simulink model "Bldc_torque_control (1)"  (R2023a)
settings: Solver=FixedStepAuto  StartTime=0.0  StopTime=2  FixedStep=5e-7  RelTol=1e-3
undefined symbols (not defined in the file): sigbuilder_block
libraries: cstblocks x14, spsIGBTDiodeLib x12, spsCurrentMeasurementLib x8, spsSeriesRLCBranchLib x6, spsVoltageMeasurementLib x6, spsabctoAlphaBetaZeroLib x6, spsDCVoltageSourceLib x2, simulink x2, spsPermanentMagnetSynchronousMachineLib x2, spsTriangleGeneratorLib x2, spspowerguiLib x2
settings Model: Creator=kiran  LastModifiedBy=ANKIT

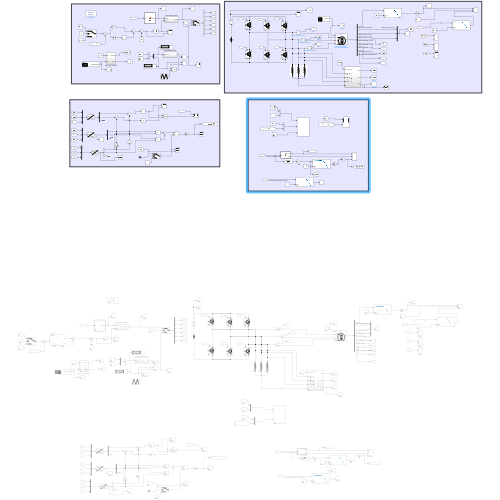
[thumbnail: Simulink's stored preview of the top-level diagram]
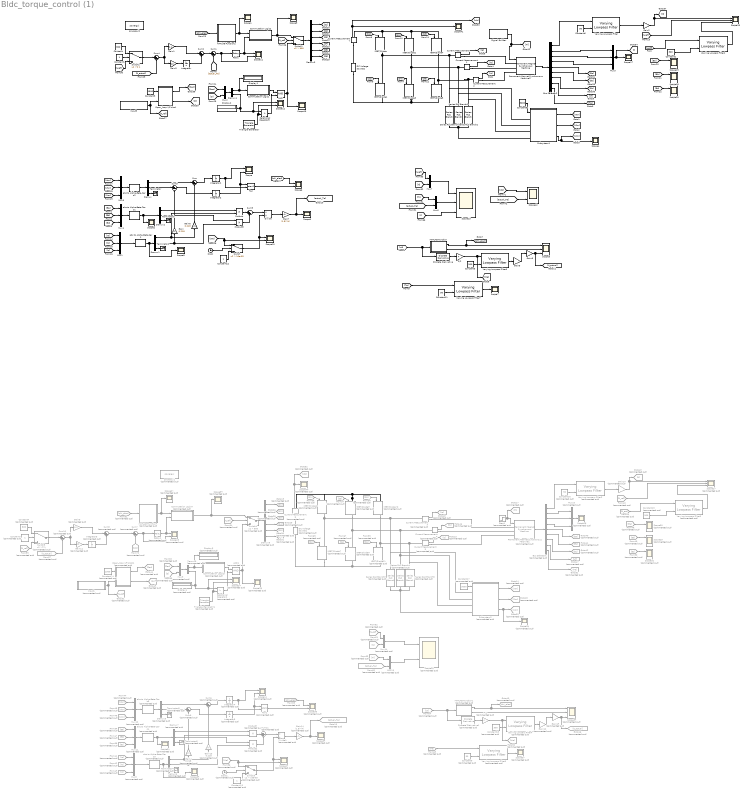
== system Bldc_torque_control (1) ==
  AND : Logic  IconShape=distinctive  AllPortsSameDT=off  OutDataTypeStr=boolean
  AND1 : Logic  Commented=on  IconShape=distinctive  AllPortsSameDT=off  OutDataTypeStr=boolean
  Bus Selector1 : BusSelector  Commented=on  OutputSignals=Rotor speed wm (rad/s),Stator current is_a (A),Stator current is_b (A),Stator current is_c (A),Stator back EMF e_a (V),Stator back EMF e_b (V),Stator back EMF e_cV),Rotor angle thetam (rad),Electromagnetic torque Te (N*m)
  Bus Selector2 : BusSelector  OutputSignals=Rotor speed wm (rad/s),Stator current is_a (A),Stator current is_b (A),Stator current is_c (A),Stator back EMF e_a (V),Stator back EMF e_b (V),Stator back EMF e_cV),Rotor angle thetam (rad),Electromagnetic torque Te (N*m)
  Clock : Clock
  Clock1 : Clock  Commented=on
  Commutation Logic1 : Subsystem
  Commutation Logic2 : Subsystem
  Commutation Logic3 : Subsystem  Commented=on
  Commutation Logic4 : Subsystem  Commented=on
  Constant : Constant  Value=800
  Constant1 : Constant
  Constant10 : Constant  Commented=on
  Constant11 : Constant  Value=50
  Constant12 : Constant
  Constant13 : Constant  Commented=on  Value=300
  Constant14 : Constant  Commented=on  Value=1500
  Constant15 : Constant  Commented=on  Value=300
  Constant16 : Constant  Commented=on  Value=50
  Constant17 : Constant  Commented=on  Value=3000
  Constant2 : Constant  Value=300
  Constant3 : Constant  Value=1500
  Constant4 : Constant  Commented=on  Value=800
  Constant5 : Constant  Value=300
  Constant6 : Constant  Value=50
  Constant7 : Constant  Commented=on
  Constant8 : Constant  Value=3000
  Constant9 : Constant  Commented=on  Value=50
  Current Measurement{,1..2,7} (4 alike) : spsCurrentMeasurementLib/Current Measurement  PhasorSimulation=off  OutputType=Complex  PSBequivalent=0
  Current Measurement{3..6} (4 alike) : spsCurrentMeasurementLib/Current Measurement  Commented=on  PhasorSimulation=off  OutputType=Complex  PSBequivalent=0
  DC Voltage Source1 : spsDCVoltageSourceLib/DC Voltage Source  Commented=on  Amplitude=33  Measurements=None
  DC Voltage Source2 : spsDCVoltageSourceLib/DC Voltage Source  Amplitude=33  Measurements=None
  Demux : Demux  Outputs=3
  Demux1 : Demux  Outputs=3
  Demux2 : Demux  Outputs=3
  Demux3 : Demux  Outputs=6
  Demux4 : Demux  Outputs=2
  Demux5 : Demux  Commented=on  Outputs=3
  Demux6 : Demux  Commented=on  Outputs=3
  Demux7 : Demux  Commented=on  Outputs=3
  Demux8 : Demux  Commented=on  Outputs=6
  Demux9 : Demux  Commented=on  Outputs=2
  Discrete Derivative : simulink/Discrete/Discrete Derivative  gainval=1.0  ICPrevScaledInput=0.0  OutMin=[]  OutMax=[]  OutDataType=fixdt(1, 16)  OutScaling=2^-10  DoSatur=off
  Discrete Derivative1 : simulink/Discrete/Discrete Derivative  Commented=on  gainval=1.0  ICPrevScaledInput=0.0  OutMin=[]  OutMax=[]  OutDataType=fixdt(1, 16)  OutScaling=2^-10  DoSatur=off
  Display1 : Display
  Display2 : Display
  Display3 : Display  Commented=on
  Display4 : Display  Commented=on
  Divide : Product  Inputs=*/
  Divide1 : Product  Commented=on  Inputs=*/
  From35 : From  Commented=on  GotoTag=N_est
  From36 : From  Commented=on  GotoTag=Ea
  From37 : From  Commented=on  GotoTag=S3
  From38 : From  Commented=on  GotoTag=S5
  From39 : From  Commented=on  GotoTag=S6
  From{40,54,59,62} (4 alike) : From  Commented=on  GotoTag=N_ref
  From41 : From  Commented=on  GotoTag=Ia
  From42 : From  Commented=on  GotoTag=Ib
  From43 : From  Commented=on  GotoTag=Ic
  From44 : From  Commented=on  GotoTag=Van
  From45 : From  Commented=on  GotoTag=Vbn
  From46 : From  Commented=on  GotoTag=Vcn
  From47 : From  Commented=on  GotoTag=Eb
  From48 : From  Commented=on  GotoTag=Ea
  From49 : From  Commented=on  GotoTag=Eb
  From50 : From  Commented=on  GotoTag=Ec
  From51 : From  Commented=on  GotoTag=phi_elec
  From52 : From  Commented=on  GotoTag=Sec
  From53 : From  Commented=on  GotoTag=D
  From55 : From  Commented=on  GotoTag=phi_elec
  From56 : From  Commented=on  GotoTag=We
  From57 : From  Commented=on  GotoTag=N_actual
  From58 : From  Commented=on  GotoTag=Ec
  From60 : From  Commented=on  GotoTag=actual_Te
  From61 : From  Commented=on  GotoTag=N
  From63 : From  Commented=on  GotoTag=Tl
  From64 : From  Commented=on  GotoTag=wt
  From65 : From  Commented=on  GotoTag=Te
  From67 : From  Commented=on  GotoTag=S4
  From68 : From  Commented=on  GotoTag=S1
  From69 : From  Commented=on  GotoTag=S2
  From70 : From  Commented=on  GotoTag=Idc
  Gain : Gain  Gain=0.218
  Gain1 : Gain  Gain=0.1
  Gain10 : Gain  Commented=on  Gain=30/pi
  Gain11 : Gain  Commented=on  Gain=10
  Gain12 : Gain  Commented=on  Gain=30/pi
  Gain13 : Gain  Commented=on  Gain=0.218
  Gain14 : Gain  Commented=on  Gain=(1.5)*(4)
  Gain15 : Gain  Commented=on  Gain=0.25
  Gain2 : Gain  Gain=30/pi
  Gain3 : Gain  Gain=10
  Gain4 : Gain  Commented=on  Gain=0.218
  Gain5 : Gain  Gain=30/pi
  Gain6 : Gain  Gain=0.218
  Gain7 : Gain  Gain=(1.5)*(4)
  Gain8 : Gain  Gain=0.25
  Gain9 : Gain  Commented=on  Gain=0.1
  Goto13 : Goto  Commented=on  GotoTag=Ic
  Goto14 : Goto  Commented=on  GotoTag=Van
  Goto15 : Goto  Commented=on  GotoTag=actual_Te
  Goto16 : Goto  Commented=on  GotoTag=N_actual
  Goto17 : Goto  Commented=on  GotoTag=Tl
  Goto18 : Goto  Commented=on  GotoTag=Vbn
  Goto19 : Goto  Commented=on  GotoTag=S1
  Goto26 : Goto  Commented=on  GotoTag=S2
  Goto28 : Goto  Commented=on  GotoTag=S3
  Goto29 : Goto  Commented=on  GotoTag=S4
  Goto30 : Goto  Commented=on  GotoTag=S5
  Goto31 : Goto  Commented=on  GotoTag=S6
  Goto32 : Goto  Commented=on  GotoTag=N_ref
  Goto33 : Goto  Commented=on  GotoTag=Vcn
  Goto40 : Goto  Commented=on  GotoTag=Ea
  Goto41 : Goto  Commented=on  GotoTag=Eb
  Goto42 : Goto  Commented=on  GotoTag=Ec
  Goto43 : Goto  Commented=on  GotoTag=N
  Goto44 : Goto  Commented=on  GotoTag=Sec
  Goto45 : Goto  Commented=on  GotoTag=D
  Goto46 : Goto  Commented=on  GotoTag=Ib
  Goto47 : Goto  Commented=on  GotoTag=wt
  Goto48 : Goto  Commented=on  GotoTag=Ia
  Goto49 : Goto  Commented=on  GotoTag=phi_elec
  Goto50 : Goto  Commented=on  GotoTag=We
  Goto51 : Goto  Commented=on  GotoTag=Te
  Goto52 : Goto  Commented=on  GotoTag=Idc
  IGBT/Diode{,1..5} (6 alike) : spsIGBTDiodeLib/IGBT//Diode  Ron=1e-3  Rs=1e5  Cs=inf  Measurements=on
  IGBT/Diode{6..11} (6 alike) : spsIGBTDiodeLib/IGBT//Diode  Commented=on  Ron=1e-3  Rs=1e5  Cs=inf  Measurements=on
  Input1 : Subsystem  Tag=STV Subsys  Commented=on  LoadFcn=sigbuilder_block('load');  StartFcn=sigbuilder_block('start');  StopFcn=sigbuilder_block('stop');  ClipboardFcn=sigbuilder_block('clipboard');  mask(Sigbuilder block){tuvar=[0:10]}
      mask help: Simulink:masks:SigbuilderBlock_MD
      mask init:
      | if ~strcmp(get_param(bdroot(gcbh),'SimulationStatus'),'stopped') tuvar = sigbuilder_block('maskInit'); end
      settings: CopyFcn=sigbuilder_block('copy');  DeleteFcn=sigbuilder_block('delete');  ModelCloseFcn=sigbuilder_block('modelClose');  PreSaveFcn=sigbuilder_block('preSave');  PauseFcn=sigbuilder_block('pause');  ContinueFcn=sigbuilder_block('continue');  NameChangeFcn=sigbuilder_block('namechange');  OpenFcn=sigbuilder_block('open',[6 36 1524 722.25 ]);  CloseFcn=sigbuilder_block('close');
      mask Display: plot(0, 0, 100, 100,[2, 2, 32, 32, 2], [68, 8, 8, 68, 68],[32, 2], [38, 38], [32, 19, 2],[53, 60, 44], [32, 17, 17, 2],[16, 16, 31, 31]);txt = getActiveGroup(gcbh);text(2, 100, txt,'verticalAlignment', 'top');
  Input3 : Subsystem  Tag=STV Subsys  LoadFcn=sigbuilder_block('load');  StartFcn=sigbuilder_block('start');  StopFcn=sigbuilder_block('stop');  ClipboardFcn=sigbuilder_block('clipboard');  mask(Sigbuilder block){tuvar=[0:10]}
      mask help: Simulink:masks:SigbuilderBlock_MD
      mask init:
      | if ~strcmp(get_param(bdroot(gcbh),'SimulationStatus'),'stopped') tuvar = sigbuilder_block('maskInit'); end
      settings: CopyFcn=sigbuilder_block('copy');  DeleteFcn=sigbuilder_block('delete');  ModelCloseFcn=sigbuilder_block('modelClose');  PreSaveFcn=sigbuilder_block('preSave');  PauseFcn=sigbuilder_block('pause');  ContinueFcn=sigbuilder_block('continue');  NameChangeFcn=sigbuilder_block('namechange');  OpenFcn=sigbuilder_block('open',[6 36 1524 722.25 ]);  CloseFcn=sigbuilder_block('close');
      mask Display: plot(0, 0, 100, 100,[2, 2, 32, 32, 2], [68, 8, 8, 68, 68],[32, 2], [38, 38], [32, 19, 2],[53, 60, 44], [32, 17, 17, 2],[16, 16, 31, 31]);txt = getActiveGroup(gcbh);text(2, 100, txt,'verticalAlignment', 'top');
  Integrator : Integrator
  Integrator1 : Integrator
  Integrator2 : Integrator
  Integrator3 : Integrator  Commented=on
  Integrator4 : Integrator  Commented=on
  Integrator5 : Integrator  Commented=on
  MATLAB Function : MATLAB Function  TreatAsAtomicUnit=on
  MATLAB Function1 : MATLAB Function  Commented=on  TreatAsAtomicUnit=on
  MATLAB Function2 : MATLAB Function  TreatAsAtomicUnit=on
  MATLAB Function3 : MATLAB Function  Commented=on  TreatAsAtomicUnit=on
  Mux{1,3..5} (4 alike) : Mux  Inputs=3
  Mux{8,10..12} (4 alike) : Mux  Commented=on  Inputs=3
  Mux13 : Mux  Commented=on  Inputs=2
  Mux14 : Mux  Commented=on  Inputs=2
  Mux2 : Mux  Inputs=2
  Mux6 : Mux  Inputs=2
  Mux7 : Mux  Inputs=2
  Mux9 : Mux  Commented=on  Inputs=2
  Open_loop V/f block : Subsystem
  Open_loop V/f block1 : Subsystem  Commented=on
  P/1 : Gain  Commented=on  Gain=4
  P/2 : Gain  Gain=4
  Permanent Magnet Synchronous Machine1 : spsPermanentMagnetSynchronousMachineLib/Permanent Magnet Synchronous Machine  Commented=on  NbPhases=3  FluxDistribution=Trapezoidal  RotorType=Round  MechanicalLoad=Torque Tm  PresetModel="05:  8 Nm 300 Vdc 2000 RPM - 10 Nm"  ShowDetailedParameters=on  MeasurementBus=off  Resistance=0.218  Inductance=0.264e-3  dqInductances=[0.0133 0.0147]  La=0.00525  MachineConstant=Voltage Constant (V_peak L-L / krpm)  Flux=0.0188  VoltageCst=15.7499  TorqueCst=0.1504  Flat=120  Mechanical=[0.00028 0.0003035 4 0]  PolePairs=4  InitialConditions=[0,0, 0,0]  InitialConditions5ph=[0 0 0 0 0 0]  RefAngle=Aligned with phase A axis (original Park)  IterativeDiscreteModel=Trapezoidal non iterative  TsBlock=-1  TsPowergui=0
  Permanent Magnet Synchronous Machine2 : spsPermanentMagnetSynchronousMachineLib/Permanent Magnet Synchronous Machine  NbPhases=3  FluxDistribution=Trapezoidal  RotorType=Round  MechanicalLoad=Torque Tm  PresetModel="05:  8 Nm 300 Vdc 2000 RPM - 10 Nm"  ShowDetailedParameters=on  MeasurementBus=off  Resistance=0.218  Inductance=0.264e-3  dqInductances=[0.0133 0.0147]  La=0.00525  MachineConstant=Voltage Constant (V_peak L-L / krpm)  Flux=0.0188  VoltageCst=15.7499  TorqueCst=0.1504  Flat=120  Mechanical=[0.00028 0.0003035 4 0]  PolePairs=4  InitialConditions=[0,0, 0,0]  InitialConditions5ph=[0 0 0 0 0 0]  RefAngle=Aligned with phase A axis (original Park)  IterativeDiscreteModel=Trapezoidal non iterative  TsBlock=-1  TsPowergui=0
  Product : Product
  Product1 : Product  Commented=on
  Product2 : Product  Commented=on
  Product3 : Product
  Relational Operator1 : RelationalOperator  Commented=on  Operator=>  OutDataTypeStr=boolean  RndMeth=Simplest  InputSameDT=off
  Relational Operator3 : RelationalOperator  Operator=>  OutDataTypeStr=boolean  RndMeth=Simplest  InputSameDT=off
  Relay : Relay  OnSwitchValue=0.05  OffSwitchValue=-0.05  OffOutputValue=-1
  Relay1 : Relay  Commented=on  OnSwitchValue=0.1  OffSwitchValue=-0.1  OffOutputValue=-1
  Scope{,6,10..12,19..20,42} (8 alike) : Scope  NumInputPorts=2
  Scope{1..2,4..5,7..9,15,17,41} (10 alike) : Scope
  Scope{3,13,16,18} (4 alike) : Scope  NumInputPorts=3
  Scope{14,22..25,30,32,36} (8 alike) : Scope  Commented=on  NumInputPorts=2
  Scope{21,26,28,31,34..35,37..40} (10 alike) : Scope  Commented=on
  Scope27 : Scope  Commented=on  NumInputPorts=3
  Scope29 : Scope  Commented=on  NumInputPorts=3
  Scope33 : Scope  Commented=on  NumInputPorts=3
  Series RLC Branch : spsSeriesRLCBranchLib/Series RLC Branch  LConnTagsString=__new0  RConnTagsString=__new0  BranchType=R  Resistance=1e06  Inductance=1e-3  SetiL0=off  InitialCurrent=0  Capacitance=1e-6  Setx0=off  InitialVoltage=0  Measurements=None
  Series RLC Branch1 : spsSeriesRLCBranchLib/Series RLC Branch  LConnTagsString=__new0  RConnTagsString=__new0  BranchType=R  Resistance=1e06  Inductance=1e-3  SetiL0=off  InitialCurrent=0  Capacitance=1e-6  Setx0=off  InitialVoltage=0  Measurements=None
  Series RLC Branch2 : spsSeriesRLCBranchLib/Series RLC Branch  LConnTagsString=__new0  RConnTagsString=__new0  BranchType=R  Resistance=1e06  Inductance=1e-3  SetiL0=off  InitialCurrent=0  Capacitance=1e-6  Setx0=off  InitialVoltage=0  Measurements=None
  Series RLC Branch3 : spsSeriesRLCBranchLib/Series RLC Branch  Commented=on  LConnTagsString=__new0  RConnTagsString=__new0  BranchType=R  Resistance=1e06  Inductance=1e-3  SetiL0=off  InitialCurrent=0  Capacitance=1e-6  Setx0=off  InitialVoltage=0  Measurements=None
  Series RLC Branch4 : spsSeriesRLCBranchLib/Series RLC Branch  Commented=on  LConnTagsString=__new0  RConnTagsString=__new0  BranchType=R  Resistance=1e06  Inductance=1e-3  SetiL0=off  InitialCurrent=0  Capacitance=1e-6  Setx0=off  InitialVoltage=0  Measurements=None
  Series RLC Branch5 : spsSeriesRLCBranchLib/Series RLC Branch  Commented=on  LConnTagsString=__new0  RConnTagsString=__new0  BranchType=R  Resistance=1e06  Inductance=1e-3  SetiL0=off  InitialCurrent=0  Capacitance=1e-6  Setx0=off  InitialVoltage=0  Measurements=None
  Signal Builder : Subsystem  Tag=STV Subsys  LoadFcn=sigbuilder_block('load');  StartFcn=sigbuilder_block('start');  StopFcn=sigbuilder_block('stop');  ClipboardFcn=sigbuilder_block('clipboard');  mask(Sigbuilder block){tuvar=[0:10]}
      mask help: Simulink:masks:SigbuilderBlock_MD
      mask init:
      | if ~strcmp(get_param(bdroot(gcbh),'SimulationStatus'),'stopped') tuvar = sigbuilder_block('maskInit'); end
      settings: CopyFcn=sigbuilder_block('copy');  DeleteFcn=sigbuilder_block('delete');  ModelCloseFcn=sigbuilder_block('modelClose');  PreSaveFcn=sigbuilder_block('preSave');  PauseFcn=sigbuilder_block('pause');  ContinueFcn=sigbuilder_block('continue');  NameChangeFcn=sigbuilder_block('namechange');  OpenFcn=sigbuilder_block('open',[0 36 1536 766.5 ]);  CloseFcn=sigbuilder_block('close');
      mask Display: plot(0, 0, 100, 100,[2, 2, 32, 32, 2], [68, 8, 8, 68, 68],[32, 2], [38, 38], [32, 19, 2],[53, 60, 44], [32, 17, 17, 2],[16, 16, 31, 31]);txt = getActiveGroup(gcbh);text(2, 100, txt,'verticalAlignment', 'top');
  Step1 : Step  Commented=on  After=0.8  SampleTime=0
  Subsystem1 : Subsystem
  Subsystem2 : Subsystem  Commented=on
  Sum{,1,3..4} (4 alike) : Sum  Inputs=|+-
  Sum{6..7,9..10} (4 alike) : Sum  Commented=on  Inputs=|+-
  Sum11 : Sum  Commented=on  Inputs=|++
  Sum2 : Sum  Inputs=|++
  Sum5 : Sum  Inputs=|++
  Sum8 : Sum  Commented=on  Inputs=|++
  Switch : Switch  Criteria=u2 > Threshold  Threshold=10e-03  SaturateOnIntegerOverflow=off  InputSameDT=off
  Switch1 : Switch  Criteria=u2 > Threshold  Threshold=900  SaturateOnIntegerOverflow=off  InputSameDT=off
  Switch2 : Switch  Threshold=1  SaturateOnIntegerOverflow=off  InputSameDT=off
  Switch3 : Switch  Commented=on  Criteria=u2 > Threshold  Threshold=10e-03  SaturateOnIntegerOverflow=off  InputSameDT=off
  Switch4 : Switch  Commented=on  Criteria=u2 > Threshold  Threshold=900  SaturateOnIntegerOverflow=off  InputSameDT=off
  Switch5 : Switch  Commented=on  Threshold=1  SaturateOnIntegerOverflow=off  InputSameDT=off
  Tan : Trigonometry  Operator=atan2
  Tan1 : Trigonometry  Commented=on  Operator=atan2
  Terminator : Terminator
  Terminator1 : Terminator
  Terminator2 : Terminator
  Terminator3 : Terminator  Commented=on
  Terminator4 : Terminator  Commented=on
  Terminator5 : Terminator  Commented=on
  Triangle Generator : spsTriangleGeneratorLib/Triangle Generator  Freq=10e3  Phase=0  Ts=0
  Triangle Generator1 : spsTriangleGeneratorLib/Triangle Generator  Commented=on  Freq=10e3  Phase=0  Ts=0
  Varying Lowpass Filter{,1,6..7} (4 alike) : cstblocks/Linear Parameter Varying/Varying Lowpass Filter  N=1
  Varying Lowpass Filter{2..5} (4 alike) : cstblocks/Linear Parameter Varying/Varying Lowpass Filter  Commented=on  N=1
  abc to Alpha-Beta-Zero : spsabctoAlphaBetaZeroLib/abc to Alpha-Beta-Zero
  abc to Alpha-Beta-Zero1 : spsabctoAlphaBetaZeroLib/abc to Alpha-Beta-Zero
  abc to Alpha-Beta-Zero2 : spsabctoAlphaBetaZeroLib/abc to Alpha-Beta-Zero
  abc to Alpha-Beta-Zero3 : spsabctoAlphaBetaZeroLib/abc to Alpha-Beta-Zero  Commented=on
  abc to Alpha-Beta-Zero4 : spsabctoAlphaBetaZeroLib/abc to Alpha-Beta-Zero  Commented=on
  abc to Alpha-Beta-Zero5 : spsabctoAlphaBetaZeroLib/abc to Alpha-Beta-Zero  Commented=on
  powergui1 : spspowerguiLib/powergui  Priority=1  Commented=on  SimulationMode=Discrete  SampleTime=1e-6  frequency=60  Iterations=50  frequencyindice=0  Pbase=100e6  ErrMax=1e-4  UnitsV=kV  UnitsW=MW  buscounter=0  FunctionMessages=off  echomessages=off  EnableUseOfTLC=off  CurrentSourceSwitches=off  DisableSnubberDevices=off  DisableRonSwitches=off  DisableVfSwitches=off  DisplayEquations=off  AutomaticDiscreteSolvers=off  SolverType=Tustin/Backward Euler (TBE)  Interpol=off  ExternalGateDelay=off  methode=off  Ts=100  x0status=blocks  SPID=on  SwTol=0  HookPort=off  NonlinearTolerance=1e-4  nMaxIteration=100  ContinueOnMaxIteration=off  RestoreLinks=warning  ResistiveCurrentMeasurement=off  Frange=[0:2:500]  Ylog=off  Xlog=on  ShowGrid=off  save=off  variable=ZData  structure=0  ZoomFFT=off  StartTime=0.0  cycles=1  DisplayStyle=1  fundamental=60  FreqAxis=off  MaxFrequency=1000  frequencyindicesteady=1  RmsSteady=1  display=off
  powergui2 : spspowerguiLib/powergui  Priority=1  SimulationMode=Discrete  SampleTime=1e-6  frequency=60  Iterations=50  frequencyindice=0  Pbase=100e6  ErrMax=1e-4  UnitsV=kV  UnitsW=MW  buscounter=0  FunctionMessages=off  echomessages=off  EnableUseOfTLC=off  CurrentSourceSwitches=off  DisableSnubberDevices=off  DisableRonSwitches=off  DisableVfSwitches=off  DisplayEquations=off  AutomaticDiscreteSolvers=off  SolverType=Tustin/Backward Euler (TBE)  Interpol=off  ExternalGateDelay=off  methode=off  Ts=100  x0status=blocks  SPID=on  SwTol=0  HookPort=off  NonlinearTolerance=1e-4  nMaxIteration=100  ContinueOnMaxIteration=off  RestoreLinks=warning  ResistiveCurrentMeasurement=off  Frange=[0:2:500]  Ylog=off  Xlog=on  ShowGrid=off  save=off  variable=ZData  structure=0  ZoomFFT=off  StartTime=0.0  cycles=1  DisplayStyle=1  fundamental=60  FreqAxis=off  MaxFrequency=1000  frequencyindicesteady=1  RmsSteady=1  display=off
  wires:
  [S1] -> IGBT/Diode/1
  Bus Selector2/3 -> Mux3/2  "<Stator current is_b (A)>"
  [Ec] -> Scope20/1
  [S5] -> IGBT/Diode4/1
  Permanent Magnet Synchronous Machine2/1 -> Bus Selector2/1
  [S2] -> IGBT/Diode1/1
  [S4] -> IGBT/Diode3/1
  Bus Selector2/2 -> Mux3/1  "<Stator current is_a (A)>"
  Constant6/1 -> Varying Lowpass Filter/2
  Bus Selector2/1 -> Varying Lowpass Filter/1  "<Rotor speed wm (rad/s)>"
  Mux3/1 -> [I], Scope17/1
  Bus Selector2/4 -> Mux3/3  "<Stator current is_c (A)>"
  Varying Lowpass Filter/1 -> Gain2/1
  Gain2/1 -> [N], Scope16/1
  [S6] -> IGBT/Diode5/1
  [Ea] -> Scope19/1
  [Eb] -> Scope18/1
  Bus Selector2/6 -> [Eb]  "<Stator back EMF e_b (V)>"
  [S3] -> IGBT/Diode2/1
  Bus Selector2/5 -> [Ea]  "<Stator back EMF e_a (V)>"
  Bus Selector2/7 -> [Ec]  "<Stator back EMF e_cV)>"
  [N_ref] -> Scope16/2
  Constant2/1 -> Varying Lowpass Filter1/2
  Varying Lowpass Filter1/1 -> Scope16/3
  [N_est] -> Varying Lowpass Filter1/1
  [Ea] -> Mux4/1
  [Eb] -> Mux4/2
  [Ec] -> Mux4/3
  Mux4/1 -> abc to Alpha-Beta-Zero1/1
  Bus Selector2/8 -> [wt]  "<Rotor angle thetam (rad)>"
  Subsystem1/2(Vbn) -> [Vbn]
  Constant8/1 -> Subsystem1/1(Cut_off_freq)
  Subsystem1/1(Van) -> [Van]
  Subsystem1/3(Vcn) -> Scope4/1, [Vcn]
  Current Measurement2/1 -> [Ic]
  Current Measurement1/1 -> [Ib]
  Current Measurement/1 -> [Ia]
  [Ia] -> Mux1/1
  Mux1/1 -> abc to Alpha-Beta-Zero/1
  [Ib] -> Mux1/2
  [Ic] -> Mux1/3
  [Vbn] -> Mux5/2
  Mux5/1 -> abc to Alpha-Beta-Zero2/1
  [Van] -> Mux5/1
  [Vcn] -> Mux5/3
  abc to Alpha-Beta-Zero2/1 -> Demux/1
  Demux/3 -> Terminator/1
  Demux/1 -> Sum/1
  Demux/2 -> Sum3/1
  Demux1/3 -> Terminator1/1
  Demux1/2 -> Product3/2, Gain/1
  Gain6/1 -> Sum/2
  Demux1/1 -> Product/2, Gain6/1
  Sum/1 -> Integrator1/1
  Sum3/1 -> Integrator2/1
  [phi_elec] -> Scope6/1
  Tan/1 -> Scope6/2
  Demux2/2 -> Product3/1
  abc to Alpha-Beta-Zero1/1 -> Demux2/1, Scope2/1
  Demux2/3 -> Terminator2/1
  Demux2/1 -> Product/1
  Product/1 -> Sum5/1
  Product3/1 -> Sum5/2
  Sum5/1 -> Divide/1
  Divide/1 -> Gain7/1
  Bus Selector2/9 -> [Te]  "<Electromagnetic torque Te (N*m)>"
  [We] -> Scope10/2, Switch/1
  Switch/1 -> Scope10/1, Divide/2
  Clock/1 -> Switch/2
  Constant12/1 -> Switch/3
  Gain7/1 -> Scope5/1, [actual_Te]
  abc to Alpha-Beta-Zero/1 -> Scope8/1, Demux1/1
  Sum2/1 -> Sum1/1
  [actual_Te] -> Sum1/2
  Sum1/1 -> Scope11/2, Relay/1
  Relay/1 -> Commutation Logic2/2(Tau), Scope11/1
  [phi_elec] -> MATLAB Function2/1(wt)
  MATLAB Function2/1(sector) -> Commutation Logic2/1(sector), Scope1/1
  Commutation Logic2/1(pulses) -> Scope9/1, Switch1/1
  Demux3/5 -> [S5]
  Demux3/2 -> [S2]
  Demux3/1 -> [S1]
  Demux3/3 -> [S3]
  Demux3/4 -> [S4]
  Switch1/1 -> Demux3/1
  Demux3/6 -> [S6]
  Demux4/1 -> Display1/1, Commutation Logic1/1(sector)
  Input3/1(RpmRequest) -> Open_loop V/f block/2(Wr), [N_ref]
  Commutation Logic1/1(Out1) -> AND/1
  [Sec] -> Mux2/1
  [D] -> Mux2/2
  Open_loop V/f block/2(Duty) -> [D]
  Open_loop V/f block/1(Sector) -> [Sec]
  Mux2/1 -> Demux4/1
  Constant3/1 -> Open_loop V/f block/1(Ws)
  Relational Operator3/1 -> AND/2
  AND/1 -> Scope15/1, Switch1/3
  Triangle Generator/1 -> Scope12/2, Relational Operator3/2
  Demux4/2 -> Display2/1, Scope12/1, Relational Operator3/1
  [N_ref] -> Switch1/2
  Integrator1/1 -> Tan/2, Scope/1
  Gain/1 -> Sum3/2
  Integrator2/1 -> Scope/2, Tan/1
  Varying Lowpass Filter7/1 -> Scope7/1
  [Te] -> Varying Lowpass Filter7/1
  Constant5/1 -> Varying Lowpass Filter6/2
  Gain8/1 -> [N_actual], Scope3/3
  MATLAB Function/2(phi) -> Scope3/2
  Discrete Derivative/1 -> P/2/1
  [wt] -> Discrete Derivative/1, MATLAB Function/1(wt)
  MATLAB Function/1(phi_elec) -> [phi_elec], Scope3/1
  Varying Lowpass Filter6/1 -> Gain5/1
  Constant11/1 -> Varying Lowpass Filter7/2
  P/2/1 -> [We], Varying Lowpass Filter6/1
  Gain5/1 -> Gain8/1
  Signal Builder/1(Signal 1) -> Permanent Magnet Synchronous Machine2/1, [Tl]
  Integrator/1 -> Sum2/2
  Gain1/1 -> Sum2/1
  [N_ref] -> Switch2/3
  Constant1/1 -> Switch2/2
  Constant/1 -> Switch2/1
  Gain3/1 -> Integrator/1
  Switch2/1 -> Sum4/1
  Sum4/1 -> Gain3/1, Gain1/1
  [N_actual] -> Sum4/2
  [actual_Te] -> Mux6/2
  [Tl] -> Mux6/1
  Mux7/1 -> Scope13/1
  Mux6/1 -> Scope13/2
  [N] -> Mux7/2
  [N_ref] -> Mux7/1
  From61/1 -> Mux14/2
  From63/1 -> Mux13/1
  Mux14/1 -> Scope25/1
  From57/1 -> Sum10/2
  Sum10/1 -> Gain11/1, Gain9/1
  Step1/1 -> Goto17/1, Permanent Magnet Synchronous Machine1/1
  Gain12/1 -> Gain15/1
  Constant7/1 -> Switch5/2
  Constant4/1 -> Switch5/1
  Demux6/3 -> Terminator4/1
  Gain11/1 -> Integrator3/1
  From55/1 -> Scope36/1
  Discrete Derivative1/1 -> P/1/1
  Mux11/1 -> abc to Alpha-Beta-Zero4/1
  MATLAB Function1/2(phi) -> Scope33/2
  Switch5/1 -> Sum10/1
  Divide1/1 -> Gain14/1
  From59/1 -> Switch5/3
  Gain9/1 -> Sum8/1
  Sum7/1 -> Scope23/2, Relay1/1
  abc to Alpha-Beta-Zero5/1 -> Demux5/1
  Demux8/6 -> Goto31/1
  AND1/1 -> Scope26/1, Switch4/3
  From51/1 -> MATLAB Function3/1(wt)
  Varying Lowpass Filter5/1 -> Scope37/1
  Demux9/2 -> Display4/1, Scope24/1, Relational Operator1/1
  P/1/1 -> Goto50/1, Varying Lowpass Filter4/1
  From64/1 -> Discrete Derivative1/1, MATLAB Function1/1(wt)
  Demux6/1 -> Product1/2, Gain13/1
  Integrator3/1 -> Sum8/2
  From60/1 -> Mux13/2
  Constant17/1 -> Subsystem2/1(Cut_off_freq)
  Bus Selector1/6 -> Goto41/1  "<Stator back EMF e_b (V)>"
  Relay1/1 -> Commutation Logic4/2(Tau), Scope23/1
  Integrator5/1 -> Scope14/2, Tan1/1
  From65/1 -> Varying Lowpass Filter5/1
  Open_loop V/f block1/2(Duty) -> Goto45/1
  From54/1 -> Switch4/2
  Gain13/1 -> Sum6/2
  Triangle Generator1/1 -> Scope24/2, Relational Operator1/2
  Varying Lowpass Filter4/1 -> Gain12/1
  Commutation Logic3/1(Out1) -> AND1/1
  Constant14/1 -> Open_loop V/f block1/1(Ws)
  Gain4/1 -> Sum9/2
  Product2/1 -> Sum11/2
  Demux8/1 -> Goto19/1
  Integrator4/1 -> Tan1/2, Scope14/1
  Varying Lowpass Filter2/1 -> Gain10/1
  From53/1 -> Mux9/2
  Input1/1(RpmRequest) -> Open_loop V/f block1/2(Wr), Goto32/1
  Commutation Logic4/1(pulses) -> Scope39/1, Switch4/1
  Bus Selector1/3 -> Mux10/2  "<Stator current is_b (A)>"
  Demux8/5 -> Goto30/1
  From69/1 -> IGBT/Diode7/1
  Switch4/1 -> Demux8/1
  From52/1 -> Mux9/1
  From35/1 -> Varying Lowpass Filter3/1
  From50/1 -> Scope32/1
  Demux9/1 -> Display3/1, Commutation Logic3/1(sector)
  From44/1 -> Mux12/1
  Open_loop V/f block1/1(Sector) -> Goto44/1
  Demux8/3 -> Goto28/1
  Sum11/1 -> Divide1/1
  Constant16/1 -> Varying Lowpass Filter2/2
  From36/1 -> Mux11/1
  From62/1 -> Mux14/1
  Gain14/1 -> Scope35/1, Goto15/1
  Bus Selector1/1 -> Varying Lowpass Filter2/1  "<Rotor speed wm (rad/s)>"
  Bus Selector1/4 -> Mux10/3  "<Stator current is_c (A)>"
  Varying Lowpass Filter3/1 -> Scope27/3
  From70/1 -> Sum7/2
  Sum8/1 -> Sum7/1
  Switch3/1 -> Scope22/1, Divide1/2
  Bus Selector1/9 -> Goto51/1  "<Electromagnetic torque Te (N*m)>"
  Demux7/1 -> Product1/1
  Constant13/1 -> Varying Lowpass Filter3/2
  abc to Alpha-Beta-Zero4/1 -> Demux7/1, Scope31/1
  From41/1 -> Mux8/1
  From42/1 -> Mux8/2
  Demux5/3 -> Terminator3/1
  Bus Selector1/5 -> Goto40/1  "<Stator back EMF e_a (V)>"
  Product1/1 -> Sum11/1
  Subsystem2/2(Vbn) -> Goto18/1
  From39/1 -> IGBT/Diode11/1
  From37/1 -> IGBT/Diode8/1
  Sum9/1 -> Integrator5/1
  Current Measurement3/1 -> Goto48/1
  From47/1 -> Mux11/2
  Sum6/1 -> Integrator4/1
  Demux6/2 -> Product2/2, Gain4/1
  Mux13/1 -> Scope25/2
  Demux7/2 -> Product2/1
  Mux12/1 -> abc to Alpha-Beta-Zero5/1
  From43/1 -> Mux8/3
  Tan1/1 -> Scope36/2
  MATLAB Function3/1(sector) -> Commutation Logic4/1(sector), Scope21/1
  Constant15/1 -> Varying Lowpass Filter4/2
  From45/1 -> Mux12/2
  Demux5/1 -> Sum6/1
  Current Measurement5/1 -> Goto13/1
  From49/1 -> Scope29/1
  Bus Selector1/7 -> Goto42/1  "<Stator back EMF e_cV)>"
  From58/1 -> Mux11/3
  From48/1 -> Scope30/1
  From40/1 -> Scope27/2
  Bus Selector1/8 -> Goto47/1  "<Rotor angle thetam (rad)>"
  Subsystem2/3(Vcn) -> Scope34/1, Goto33/1
  Demux5/2 -> Sum9/1
  Constant10/1 -> Switch3/3
  From68/1 -> IGBT/Diode6/1
  Demux7/3 -> Terminator5/1
  Mux8/1 -> abc to Alpha-Beta-Zero3/1
  Gain15/1 -> Goto16/1, Scope33/3
  Subsystem2/1(Van) -> Goto14/1
  Mux9/1 -> Demux9/1
  From56/1 -> Scope22/2, Switch3/1
  From38/1 -> IGBT/Diode10/1
  Mux10/1 -> Scope28/1
  Demux8/4 -> Goto29/1
  From67/1 -> IGBT/Diode9/1
  From46/1 -> Mux12/3
  Gain10/1 -> Goto43/1, Scope27/1
  abc to Alpha-Beta-Zero3/1 -> Scope38/1, Demux6/1
  Constant9/1 -> Varying Lowpass Filter5/2
  Clock1/1 -> Switch3/2
  Bus Selector1/2 -> Mux10/1  "<Stator current is_a (A)>"
  Relational Operator1/1 -> AND1/2
  Permanent Magnet Synchronous Machine1/1 -> Bus Selector1/1
  MATLAB Function1/1(phi_elec) -> Goto49/1, Scope33/1
  Current Measurement4/1 -> Goto46/1
  Demux8/2 -> Goto26/1
  Current Measurement6/1 -> Goto52/1, Scope40/1
  Current Measurement7/1 -> [Idc], Scope41/1
  [I] -> Scope13/3
  [Idc] -> Scope42/1
  [actual_Te] -> Scope42/2
  connections:
  IGBT/Diode3/RConn1 -- IGBT/Diode1/RConn1 -- DC Voltage Source2/LConn1 -- IGBT/Diode5/RConn1
  IGBT/Diode2/RConn1 -- Series RLC Branch1/LConn1 -- Subsystem1/LConn2 -- Current Measurement1/LConn1 -- IGBT/Diode3/LConn1
  IGBT/Diode/LConn1 -- IGBT/Diode4/LConn1 -- IGBT/Diode2/LConn1 -- Current Measurement7/RConn1
  IGBT/Diode/RConn1 -- Series RLC Branch/LConn1 -- Subsystem1/LConn1 -- Current Measurement/LConn1 -- IGBT/Diode1/LConn1
  IGBT/Diode4/RConn1 -- Subsystem1/LConn3 -- Series RLC Branch2/LConn1 -- Current Measurement2/LConn1 -- IGBT/Diode5/LConn1
  Current Measurement/RConn1 -- Permanent Magnet Synchronous Machine2/LConn1
  Current Measurement1/RConn1 -- Permanent Magnet Synchronous Machine2/LConn2
  Current Measurement2/RConn1 -- Permanent Magnet Synchronous Machine2/LConn3
  Series RLC Branch/RConn1 -- Series RLC Branch2/RConn1 -- Subsystem1/LConn4 -- Series RLC Branch1/RConn1
  Current Measurement5/LConn1 -- IGBT/Diode10/RConn1 -- IGBT/Diode11/LConn1 -- Subsystem2/LConn3 -- Series RLC Branch5/LConn1
  Current Measurement3/LConn1 -- IGBT/Diode6/RConn1 -- IGBT/Diode7/LConn1 -- Series RLC Branch3/LConn1 -- Subsystem2/LConn1
  Subsystem2/LConn2 -- IGBT/Diode8/RConn1 -- IGBT/Diode9/LConn1 -- Current Measurement4/LConn1 -- Series RLC Branch4/LConn1
  IGBT/Diode8/LConn1 -- Current Measurement6/RConn1 -- IGBT/Diode6/LConn1 -- IGBT/Diode10/LConn1
  IGBT/Diode11/RConn1 -- IGBT/Diode9/RConn1 -- IGBT/Diode7/RConn1 -- DC Voltage Source1/LConn1
  Series RLC Branch4/RConn1 -- Series RLC Branch3/RConn1 -- Series RLC Branch5/RConn1 -- Subsystem2/LConn4
  Current Measurement3/RConn1 -- Permanent Magnet Synchronous Machine1/LConn1
  Current Measurement5/RConn1 -- Permanent Magnet Synchronous Machine1/LConn3
  Current Measurement4/RConn1 -- Permanent Magnet Synchronous Machine1/LConn2
  DC Voltage Source1/RConn1 -- Current Measurement6/LConn1
  Current Measurement7/LConn1 -- DC Voltage Source2/RConn1

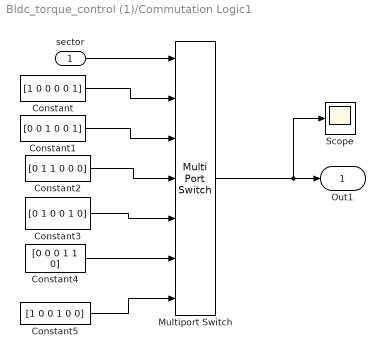
== system Bldc_torque_control (1)/Commutation Logic1 ==
  sector : Inport
  Constant : Constant  Value=[1 0 0 0 0 1]  VectorParams1D=off
  Constant1 : Constant  Value=[0 0 1 0 0 1]  VectorParams1D=off
  Constant2 : Constant  Value=[0 1 1 0 0 0]  VectorParams1D=off
  Constant3 : Constant  Value=[0 1 0 0 1 0]  VectorParams1D=off
  Constant4 : Constant  Value=[0 0 0 1 1 0]  VectorParams1D=off
  Constant5 : Constant  Value=[1 0 0 1 0 0]  VectorParams1D=off
  Multiport Switch : MultiPortSwitch  DataPortOrder=Zero-based contiguous  Inputs=6  zeroidx=on  SaturateOnIntegerOverflow=off  InputSameDT=off
  Scope : Scope
  Out1 : Outport
  wires:
  sector/1 -> Multiport Switch/1
  Multiport Switch/1 -> Scope/1, Out1/1
  Constant5/1 -> Multiport Switch/7
  Constant4/1 -> Multiport Switch/6
  Constant/1 -> Multiport Switch/2
  Constant1/1 -> Multiport Switch/3
  Constant2/1 -> Multiport Switch/4
  Constant3/1 -> Multiport Switch/5

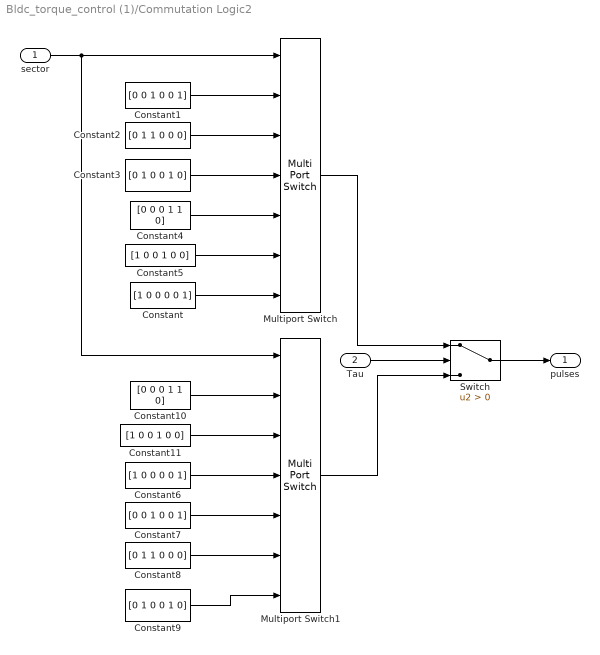
== system Bldc_torque_control (1)/Commutation Logic2 ==
  sector : Inport
  Tau : Inport  Port=2
  Constant : Constant  Value=[1 0 0 0 0 1]  VectorParams1D=off
  Constant1 : Constant  Value=[0 0 1 0 0 1]  VectorParams1D=off
  Constant10 : Constant  Value=[0 0 0 1 1 0]  VectorParams1D=off
  Constant11 : Constant  Value=[1 0 0 1 0 0]  VectorParams1D=off
  Constant2 : Constant  Value=[0 1 1 0 0 0]  VectorParams1D=off
  Constant3 : Constant  Value=[0 1 0 0 1 0]  VectorParams1D=off
  Constant4 : Constant  Value=[0 0 0 1 1 0]  VectorParams1D=off
  Constant5 : Constant  Value=[1 0 0 1 0 0]  VectorParams1D=off
  Constant6 : Constant  Value=[1 0 0 0 0 1]  VectorParams1D=off
  Constant7 : Constant  Value=[0 0 1 0 0 1]  VectorParams1D=off
  Constant8 : Constant  Value=[0 1 1 0 0 0]  VectorParams1D=off
  Constant9 : Constant  Value=[0 1 0 0 1 0]  VectorParams1D=off
  Multiport Switch : MultiPortSwitch  DataPortOrder=Zero-based contiguous  Inputs=6  zeroidx=on  SaturateOnIntegerOverflow=off  InputSameDT=off
  Multiport Switch1 : MultiPortSwitch  DataPortOrder=Zero-based contiguous  Inputs=6  zeroidx=on  SaturateOnIntegerOverflow=off  InputSameDT=off
  Switch : Switch  Criteria=u2 > Threshold  SaturateOnIntegerOverflow=off  InputSameDT=off
  pulses : Outport
  wires:
  Multiport Switch/1 -> Switch/1
  Constant/1 -> Multiport Switch/7
  Constant5/1 -> Multiport Switch/6
  Constant1/1 -> Multiport Switch/2
  Constant2/1 -> Multiport Switch/3
  Constant3/1 -> Multiport Switch/4
  Constant4/1 -> Multiport Switch/5
  Constant11/1 -> Multiport Switch1/3
  Constant7/1 -> Multiport Switch1/5
  sector/1 -> Multiport Switch/1, Multiport Switch1/1
  Multiport Switch1/1 -> Switch/3
  Constant6/1 -> Multiport Switch1/4
  Constant8/1 -> Multiport Switch1/6
  Constant10/1 -> Multiport Switch1/2
  Constant9/1 -> Multiport Switch1/7
  Tau/1 -> Switch/2
  Switch/1 -> pulses/1

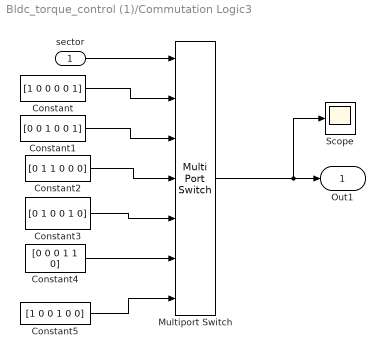
== system Bldc_torque_control (1)/Commutation Logic3 ==
  sector : Inport
  Constant : Constant  Value=[1 0 0 0 0 1]  VectorParams1D=off
  Constant1 : Constant  Value=[0 0 1 0 0 1]  VectorParams1D=off
  Constant2 : Constant  Value=[0 1 1 0 0 0]  VectorParams1D=off
  Constant3 : Constant  Value=[0 1 0 0 1 0]  VectorParams1D=off
  Constant4 : Constant  Value=[0 0 0 1 1 0]  VectorParams1D=off
  Constant5 : Constant  Value=[1 0 0 1 0 0]  VectorParams1D=off
  Multiport Switch : MultiPortSwitch  DataPortOrder=Zero-based contiguous  Inputs=6  zeroidx=on  SaturateOnIntegerOverflow=off  InputSameDT=off
  Scope : Scope
  Out1 : Outport
  wires:
  sector/1 -> Multiport Switch/1
  Multiport Switch/1 -> Scope/1, Out1/1
  Constant5/1 -> Multiport Switch/7
  Constant4/1 -> Multiport Switch/6
  Constant/1 -> Multiport Switch/2
  Constant1/1 -> Multiport Switch/3
  Constant2/1 -> Multiport Switch/4
  Constant3/1 -> Multiport Switch/5

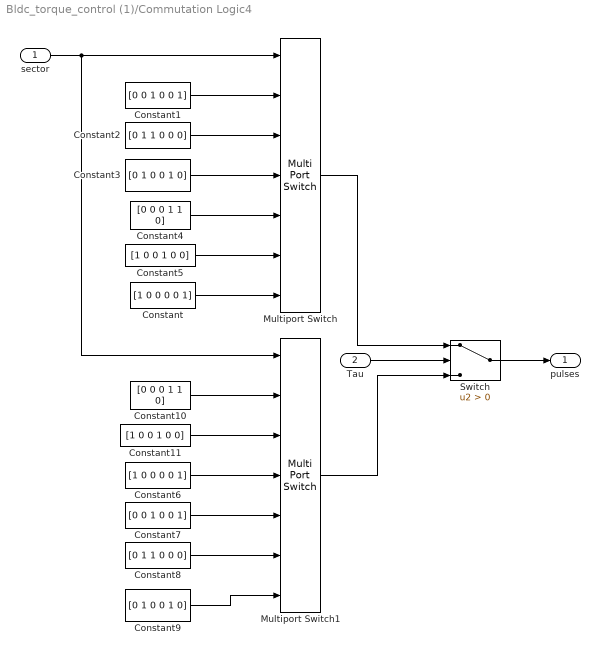
== system Bldc_torque_control (1)/Commutation Logic4 ==
  sector : Inport
  Tau : Inport  Port=2
  Constant : Constant  Value=[1 0 0 0 0 1]  VectorParams1D=off
  Constant1 : Constant  Value=[0 0 1 0 0 1]  VectorParams1D=off
  Constant10 : Constant  Value=[0 0 0 1 1 0]  VectorParams1D=off
  Constant11 : Constant  Value=[1 0 0 1 0 0]  VectorParams1D=off
  Constant2 : Constant  Value=[0 1 1 0 0 0]  VectorParams1D=off
  Constant3 : Constant  Value=[0 1 0 0 1 0]  VectorParams1D=off
  Constant4 : Constant  Value=[0 0 0 1 1 0]  VectorParams1D=off
  Constant5 : Constant  Value=[1 0 0 1 0 0]  VectorParams1D=off
  Constant6 : Constant  Value=[1 0 0 0 0 1]  VectorParams1D=off
  Constant7 : Constant  Value=[0 0 1 0 0 1]  VectorParams1D=off
  Constant8 : Constant  Value=[0 1 1 0 0 0]  VectorParams1D=off
  Constant9 : Constant  Value=[0 1 0 0 1 0]  VectorParams1D=off
  Multiport Switch : MultiPortSwitch  DataPortOrder=Zero-based contiguous  Inputs=6  zeroidx=on  SaturateOnIntegerOverflow=off  InputSameDT=off
  Multiport Switch1 : MultiPortSwitch  DataPortOrder=Zero-based contiguous  Inputs=6  zeroidx=on  SaturateOnIntegerOverflow=off  InputSameDT=off
  Switch : Switch  Criteria=u2 > Threshold  SaturateOnIntegerOverflow=off  InputSameDT=off
  pulses : Outport
  wires:
  Multiport Switch/1 -> Switch/1
  Constant/1 -> Multiport Switch/7
  Constant5/1 -> Multiport Switch/6
  Constant1/1 -> Multiport Switch/2
  Constant2/1 -> Multiport Switch/3
  Constant3/1 -> Multiport Switch/4
  Constant4/1 -> Multiport Switch/5
  Constant11/1 -> Multiport Switch1/3
  Constant7/1 -> Multiport Switch1/5
  sector/1 -> Multiport Switch/1, Multiport Switch1/1
  Multiport Switch1/1 -> Switch/3
  Constant6/1 -> Multiport Switch1/4
  Constant8/1 -> Multiport Switch1/6
  Constant10/1 -> Multiport Switch1/2
  Constant9/1 -> Multiport Switch1/7
  Tau/1 -> Switch/2
  Switch/1 -> pulses/1

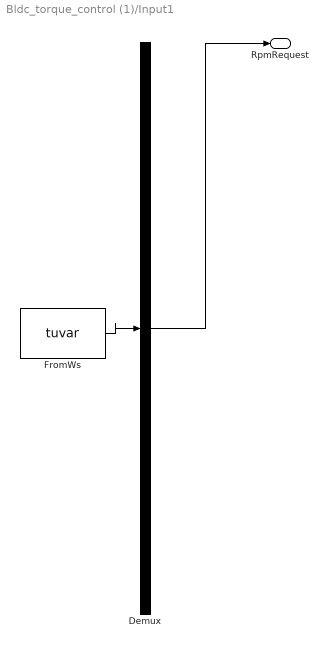
== system Bldc_torque_control (1)/Input1 ==
  Demux : Demux  Tag=STV Demux  Outputs=1
      settings: DisplayOption=none
  FromWs : FromWorkspace  Tag=STV FromWs  VariableName=tuvar
      SigBuilderData=|
      | common.afterFinalStr = 'Extrapolate'
      | common.sampleTime = 0
      | dataSet.timeRange = [0 1]
      | dataSet.name = 'Test 1'
      | sbobj.Groups.Name = 'Test 1'
      | sbobj.Groups.Signals.Name = 'RpmRequest'
      | sbobj.Groups.Signals.XData = [0 0.102 0.2 0.2 0.4 0.4 0.6 0.6 0.826 0.926 1]
      | sbobj.Groups.Signals.YData = [499 497 499 650 650 975 975 1100 1100 1102 1103]
      | sbobj.Groups.TimeRange = [0 1]
  RpmRequest : Outport  Tag=STV Outport  VectorParamsAs1DForOutWhenUnconnected=off
  wires:
  FromWs/1 -> Demux/1
  Demux/1 -> RpmRequest/1

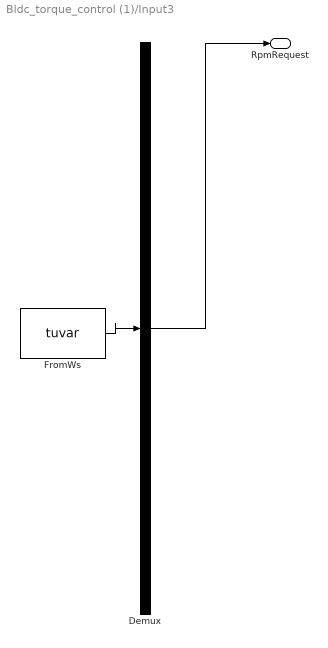
== system Bldc_torque_control (1)/Input3 ==
  Demux : Demux  Tag=STV Demux  Outputs=1
      settings: DisplayOption=none
  FromWs : FromWorkspace  Tag=STV FromWs  VariableName=tuvar
      SigBuilderData=|
      | common.afterFinalStr = 'Extrapolate'
      | common.sampleTime = 0
      | dataSet.timeRange = [0 1]
      | dataSet.name = 'Test 1'
      | sbobj.Groups.Name = 'Test 1'
      | sbobj.Groups.Signals.Name = 'RpmRequest'
      | sbobj.Groups.Signals.XData = [0 0.102 0.2 0.2 0.4 0.4 0.6 0.6 0.826 0.926 1]
      | sbobj.Groups.Signals.YData = [499 497 499 650 650 975 975 1100 1100 1102 1103]
      | sbobj.Groups.TimeRange = [0 1]
  RpmRequest : Outport  Tag=STV Outport  VectorParamsAs1DForOutWhenUnconnected=off
  wires:
  FromWs/1 -> Demux/1
  Demux/1 -> RpmRequest/1

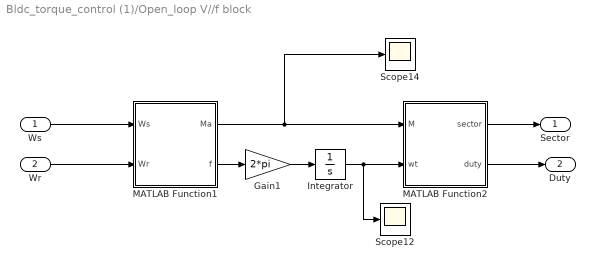
== system Bldc_torque_control (1)/Open_loop V//f block ==
  Ws : Inport
  Wr : Inport  Port=2
  Gain1 : Gain  Gain=2*pi
  Integrator : Integrator
  MATLAB Function1 : MATLAB Function  TreatAsAtomicUnit=on
  MATLAB Function2 : MATLAB Function  TreatAsAtomicUnit=on
  Scope12 : Scope
  Scope14 : Scope
  Sector : Outport  VectorParamsAs1DForOutWhenUnconnected=off
  Duty : Outport  Port=2  VectorParamsAs1DForOutWhenUnconnected=off
  wires:
  Integrator/1 -> Scope12/1, MATLAB Function2/2(wt)
  MATLAB Function1/1(Ma) -> Scope14/1, MATLAB Function2/1(M)
  MATLAB Function1/2(f) -> Gain1/1
  Gain1/1 -> Integrator/1
  Ws/1 -> MATLAB Function1/1(Ws)
  MATLAB Function2/1(sector) -> Sector/1
  MATLAB Function2/2(duty) -> Duty/1
  Wr/1 -> MATLAB Function1/2(Wr)

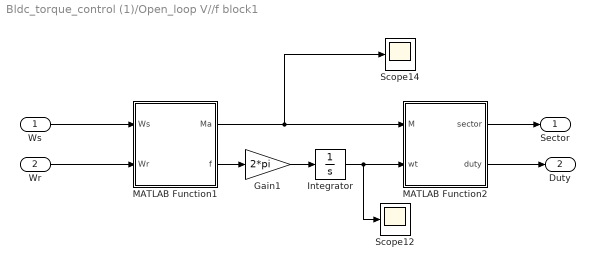
== system Bldc_torque_control (1)/Open_loop V//f block1 ==
  Ws : Inport
  Wr : Inport  Port=2
  Gain1 : Gain  Gain=2*pi
  Integrator : Integrator
  MATLAB Function1 : MATLAB Function  TreatAsAtomicUnit=on
  MATLAB Function2 : MATLAB Function  TreatAsAtomicUnit=on
  Scope12 : Scope
  Scope14 : Scope
  Sector : Outport  VectorParamsAs1DForOutWhenUnconnected=off
  Duty : Outport  Port=2  VectorParamsAs1DForOutWhenUnconnected=off
  wires:
  Integrator/1 -> Scope12/1, MATLAB Function2/2(wt)
  MATLAB Function1/1(Ma) -> Scope14/1, MATLAB Function2/1(M)
  MATLAB Function1/2(f) -> Gain1/1
  Gain1/1 -> Integrator/1
  Ws/1 -> MATLAB Function1/1(Ws)
  MATLAB Function2/1(sector) -> Sector/1
  MATLAB Function2/2(duty) -> Duty/1
  Wr/1 -> MATLAB Function1/2(Wr)

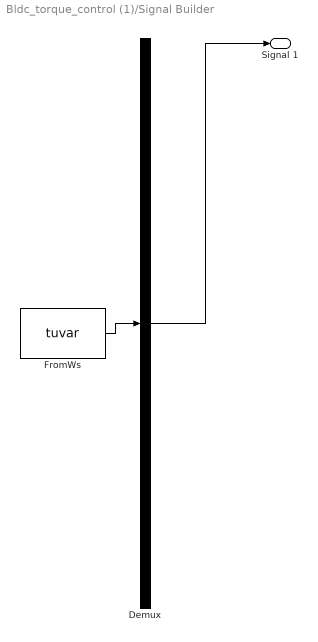
== system Bldc_torque_control (1)/Signal Builder ==
  Demux : Demux  Tag=STV Demux  Outputs=1
      settings: DisplayOption=none
  FromWs : FromWorkspace  Tag=STV FromWs  VariableName=tuvar
      SigBuilderData=|
      | common.afterFinalStr = 'Extrapolate'
      | common.sampleTime = 0
      | dataSet.timeRange = [0 3]
      | dataSet.name = 'Group 1'
      | sbobj.Groups.Name = 'Group 1'
      | sbobj.Groups.Signals.Name = 'Signal 1'
      | sbobj.Groups.Signals.XData = [0 1 1 1.498 1.498 3]
      | sbobj.Groups.Signals.YData = [0 0 0.5 0.5 -0.5 -0.5]
      | sbobj.Groups.TimeRange = [0 3]
  Signal 1 : Outport  Tag=STV Outport
  wires:
  Demux/1 -> Signal 1/1
  FromWs/1 -> Demux/1

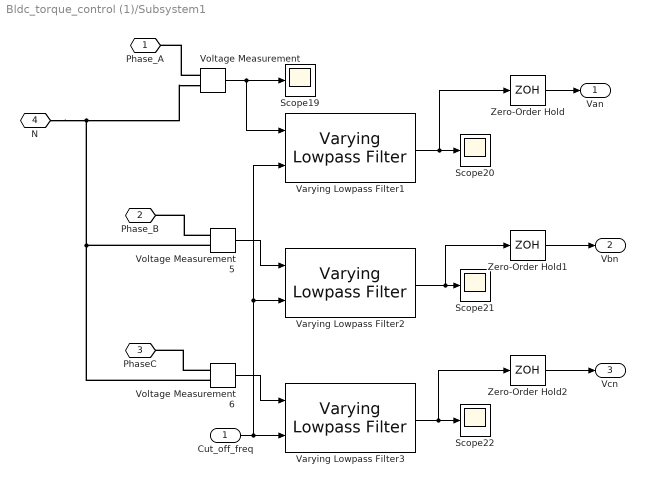
== system Bldc_torque_control (1)/Subsystem1 ==
  Cut_off_freq : Inport
  Scope{19..22} (4 alike) : Scope
  Varying Lowpass Filter1 : cstblocks/Linear Parameter Varying/Varying Lowpass Filter  N=1
  Varying Lowpass Filter2 : cstblocks/Linear Parameter Varying/Varying Lowpass Filter  N=1
  Varying Lowpass Filter3 : cstblocks/Linear Parameter Varying/Varying Lowpass Filter  N=1
  Voltage Measurement : spsVoltageMeasurementLib/Voltage Measurement  PhasorSimulation=off  OutputType=Complex  PSBequivalent=0
  Voltage Measurement5 : spsVoltageMeasurementLib/Voltage Measurement  PhasorSimulation=off  OutputType=Complex  PSBequivalent=0
  Voltage Measurement6 : spsVoltageMeasurementLib/Voltage Measurement  PhasorSimulation=off  OutputType=Complex  PSBequivalent=0
  Zero-Order Hold : ZeroOrderHold  SampleTime=-1
  Zero-Order Hold1 : ZeroOrderHold  SampleTime=-1
  Zero-Order Hold2 : ZeroOrderHold  SampleTime=-1
  Phase_A : PMIOPort  Side=Left
  Phase_B : PMIOPort  Port=2  Side=Left
  PhaseC : PMIOPort  Port=3  Side=Left
  N : PMIOPort  Port=4  Side=Left
  Van : Outport  VectorParamsAs1DForOutWhenUnconnected=off
  Vbn : Outport  Port=2  VectorParamsAs1DForOutWhenUnconnected=off
  Vcn : Outport  Port=3  VectorParamsAs1DForOutWhenUnconnected=off
  wires:
  Varying Lowpass Filter1/1 -> Zero-Order Hold/1, Scope20/1
  Varying Lowpass Filter3/1 -> Zero-Order Hold2/1, Scope22/1
  Voltage Measurement5/1 -> Varying Lowpass Filter2/1
  Voltage Measurement6/1 -> Varying Lowpass Filter3/1
  Varying Lowpass Filter2/1 -> Zero-Order Hold1/1, Scope21/1
  Voltage Measurement/1 -> Varying Lowpass Filter1/1, Scope19/1
  Cut_off_freq/1 -> Varying Lowpass Filter1/2, Varying Lowpass Filter2/2, Varying Lowpass Filter3/2
  Zero-Order Hold/1 -> Van/1
  Zero-Order Hold1/1 -> Vbn/1
  Zero-Order Hold2/1 -> Vcn/1
  connections:
  Voltage Measurement5/LConn1 -- Phase_B/RConn1
  Voltage Measurement6/LConn1 -- PhaseC/RConn1
  Voltage Measurement/LConn1 -- Phase_A/RConn1
  N/RConn1 -- Voltage Measurement6/LConn2 -- Voltage Measurement5/LConn2 -- Voltage Measurement/LConn2

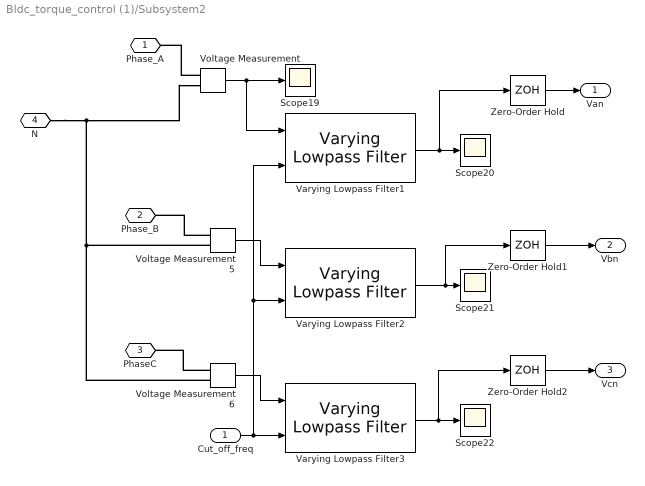
== system Bldc_torque_control (1)/Subsystem2 ==
  Cut_off_freq : Inport
  Scope{19..22} (4 alike) : Scope
  Varying Lowpass Filter1 : cstblocks/Linear Parameter Varying/Varying Lowpass Filter  N=1
  Varying Lowpass Filter2 : cstblocks/Linear Parameter Varying/Varying Lowpass Filter  N=1
  Varying Lowpass Filter3 : cstblocks/Linear Parameter Varying/Varying Lowpass Filter  N=1
  Voltage Measurement : spsVoltageMeasurementLib/Voltage Measurement  PhasorSimulation=off  OutputType=Complex  PSBequivalent=0
  Voltage Measurement5 : spsVoltageMeasurementLib/Voltage Measurement  PhasorSimulation=off  OutputType=Complex  PSBequivalent=0
  Voltage Measurement6 : spsVoltageMeasurementLib/Voltage Measurement  PhasorSimulation=off  OutputType=Complex  PSBequivalent=0
  Zero-Order Hold : ZeroOrderHold  SampleTime=-1
  Zero-Order Hold1 : ZeroOrderHold  SampleTime=-1
  Zero-Order Hold2 : ZeroOrderHold  SampleTime=-1
  Phase_A : PMIOPort  Side=Left
  Phase_B : PMIOPort  Port=2  Side=Left
  PhaseC : PMIOPort  Port=3  Side=Left
  N : PMIOPort  Port=4  Side=Left
  Van : Outport  VectorParamsAs1DForOutWhenUnconnected=off
  Vbn : Outport  Port=2  VectorParamsAs1DForOutWhenUnconnected=off
  Vcn : Outport  Port=3  VectorParamsAs1DForOutWhenUnconnected=off
  wires:
  Varying Lowpass Filter1/1 -> Zero-Order Hold/1, Scope20/1
  Varying Lowpass Filter3/1 -> Zero-Order Hold2/1, Scope22/1
  Voltage Measurement5/1 -> Varying Lowpass Filter2/1
  Voltage Measurement6/1 -> Varying Lowpass Filter3/1
  Varying Lowpass Filter2/1 -> Zero-Order Hold1/1, Scope21/1
  Voltage Measurement/1 -> Varying Lowpass Filter1/1, Scope19/1
  Cut_off_freq/1 -> Varying Lowpass Filter1/2, Varying Lowpass Filter2/2, Varying Lowpass Filter3/2
  Zero-Order Hold/1 -> Van/1
  Zero-Order Hold1/1 -> Vbn/1
  Zero-Order Hold2/1 -> Vcn/1
  connections:
  Voltage Measurement5/LConn1 -- Phase_B/RConn1
  Voltage Measurement6/LConn1 -- PhaseC/RConn1
  Voltage Measurement/LConn1 -- Phase_A/RConn1
  N/RConn1 -- Voltage Measurement6/LConn2 -- Voltage Measurement5/LConn2 -- Voltage Measurement/LConn2

== matlab function Bldc_torque_control (1)/MATLAB Function ==
  data: wt input; phi_elec output; phi output
function [phi_elec, phi] = fcn(wt)
%mechanical__angle
x = (wt/6.28);
y = floor(x);
phi = wt - (y*6.28);

% electrical__angle
theta_elec = (4)*phi;
xx = (theta_elec/6.28);
z = floor(xx);
phi_elec = theta_elec-(z*6.28);

== matlab function Bldc_torque_control (1)/Open_loop V//f block/MATLAB Function1 ==
  data: Ws input; Ma output; Wr input; f output
function [Ma,f] = fcn(Ws,Wr)
Ma=1*(Wr/Ws);
f=100*(Wr/Ws);
%f=250*(Wr/Ws);
end

== matlab function Bldc_torque_control (1)/Open_loop V//f block/MATLAB Function2 ==
  data: M input; sector output; wt input; duty output
function [sector, duty] = fcn(M,wt)
x = (wt/6.28);
y = floor(x);
theta = wt - (y*6.28);
sector = floor(theta/(pi/3));
duty = M;
end

== matlab function Bldc_torque_control (1)/MATLAB Function2 ==
  data: sector output; wt input
function sector  = fcn(wt)
x = (wt/6.28);
y = floor(x);
theta = wt - (y*6.28);
sector = floor(theta/(pi/3));
%duty = M;
end

== matlab function Bldc_torque_control (1)/MATLAB Function1 ==
  data: wt input; phi_elec output; phi output
function [phi_elec, phi] = fcn(wt)
%mechanical__angle
x = (wt/6.28);
y = floor(x);
phi = wt - (y*6.28);

% electrical__angle
theta_elec = (4)*phi;
xx = (theta_elec/6.28);
z = floor(xx);
phi_elec = theta_elec-(z*6.28);

== matlab function Bldc_torque_control (1)/MATLAB Function3 ==
  data: sector output; wt input
function sector  = fcn(wt)
x = (wt/6.28);
y = floor(x);
theta = wt - (y*6.28);
sector = floor(theta/(pi/3));
%duty = M;
end

== matlab function Bldc_torque_control (1)/Open_loop V//f block1/MATLAB Function1 ==
  data: Ws input; Ma output; Wr input; f output
function [Ma,f] = fcn(Ws,Wr)
Ma=1*(Wr/Ws);
f=100*(Wr/Ws);
%f=250*(Wr/Ws);
end

== matlab function Bldc_torque_control (1)/Open_loop V//f block1/MATLAB Function2 ==
  data: M input; sector output; wt input; duty output
function [sector, duty] = fcn(M,wt)
x = (wt/6.28);
y = floor(x);
theta = wt - (y*6.28);
sector = floor(theta/(pi/3));
duty = M;
end
